simulink model "rcmodel"  (R2024b)
settings: Solver=FixedStepAuto  StartTime=0.0  StopTime=3500  FixedStep=0.1  RelTol=1e-3
undefined symbols (not defined in the file): ocv_interp, soc_target
libraries: fl_lib x8, nesl_utility x5, spspowerguiLib x1
settings Model: Creator=Acer  LastModifiedBy=Acer

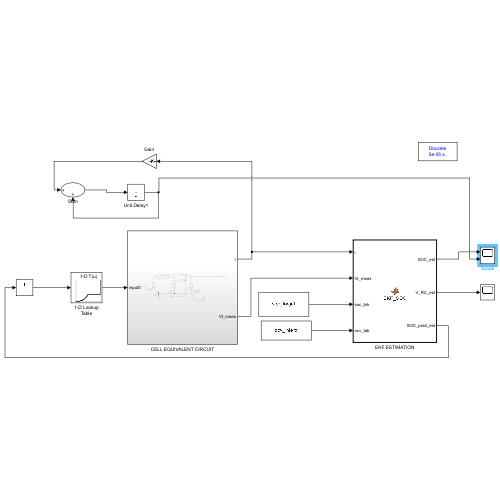
[thumbnail: Simulink's stored preview of the top-level diagram]
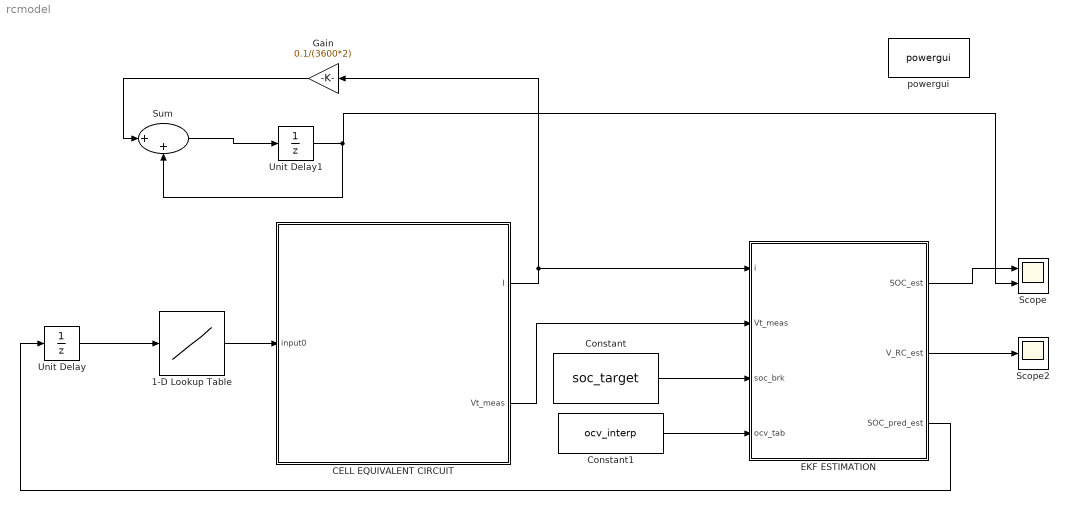
== system rcmodel ==
  1-D Lookup Table : Lookup_n-D  NumberOfTableDimensions=1  BreakpointsForDimension1=soc_target  Table=ocv_interp  ExtrapMethod=Clip  InternalRulePriority=Speed  RndMeth=Simplest
  CELL EQUIVALENT CIRCUIT : Subsystem
  Constant : Constant  Value=soc_target  SampleTime=0.1
  Constant1 : Constant  Value=ocv_interp  SampleTime=0.1
  EKF ESTIMATION : MATLAB Function  TreatAsAtomicUnit=on
  Gain : Gain  Gain=0.1/(3600*2)
  Scope : Scope  NumInputPorts=2
  Scope2 : Scope
  Sum : Sum  Inputs=|++
  Unit Delay : UnitDelay  InitialCondition=1  SampleTime=0.1  HasFrameUpgradeWarning=on
  Unit Delay1 : UnitDelay  InitialCondition=1  SampleTime=-1  HasFrameUpgradeWarning=on
  powergui : spspowerguiLib/powergui  Priority=1  SimulationMode=Discrete  SampleTime=50e-6  frequency=60  Iterations=50  frequencyindice=0  Pbase=100e6  ErrMax=1e-4  UnitsV=kV  UnitsW=MW  buscounter=0  FunctionMessages=off  echomessages=off  EnableUseOfTLC=off  CurrentSourceSwitches=off  DisableSnubberDevices=off  DisableRonSwitches=off  DisableVfSwitches=off  DisplayEquations=off  AutomaticDiscreteSolvers=off  SolverType=Tustin/Backward Euler (TBE)  Interpol=off  ExternalGateDelay=off  methode=off  Ts=100  x0status=blocks  SPID=on  SwTol=0  HookPort=off  NonlinearTolerance=1e-4  nMaxIteration=100  ContinueOnMaxIteration=off  RestoreLinks=warning  ResistiveCurrentMeasurement=off  Frange=[0:2:500]  Ylog=off  Xlog=on  ShowGrid=off  save=off  variable=ZData  structure=0  ZoomFFT=off  StartTime=0.0  cycles=1  DisplayStyle=1  fundamental=60  FreqAxis=off  MaxFrequency=1000  frequencyindicesteady=1  RmsSteady=1  display=off
  wires:
  Constant/1 -> EKF ESTIMATION/3(soc_brk)
  Constant1/1 -> EKF ESTIMATION/4(ocv_tab)
  EKF ESTIMATION/2(V_RC_est) -> Scope2/1
  Unit Delay1/1 -> Scope/2, Sum/2
  EKF ESTIMATION/1(SOC_est) -> Scope/1
  Unit Delay/1 -> 1-D Lookup Table/1
  EKF ESTIMATION/3(SOC_pred_est) -> Unit Delay/1
  Sum/1 -> Unit Delay1/1
  Gain/1 -> Sum/1
  CELL EQUIVALENT CIRCUIT/1(I) -> Gain/1, EKF ESTIMATION/1(i)
  1-D Lookup Table/1 -> CELL EQUIVALENT CIRCUIT/1(input0)
  CELL EQUIVALENT CIRCUIT/2(Vt_meas) -> EKF ESTIMATION/2(Vt_meas)

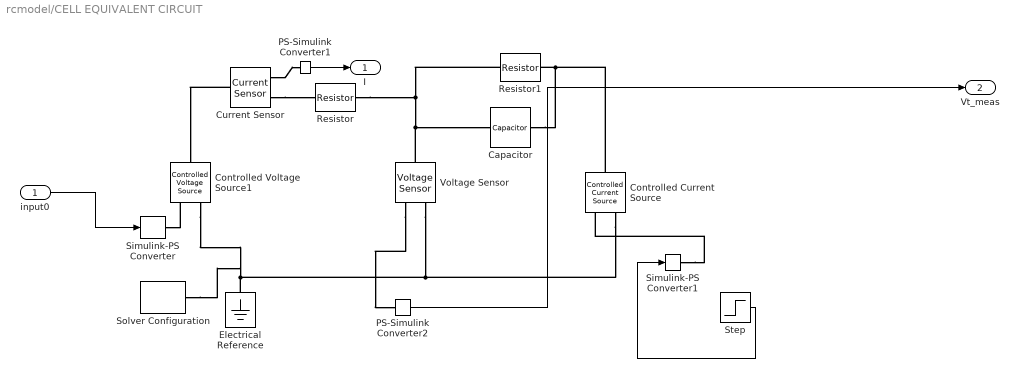
== system rcmodel/CELL EQUIVALENT CIRCUIT ==
  input0 : Inport
  Capacitor : fl_lib/Electrical/Electrical Elements/Capacitor  c=540 F  r=0 Ohm  g=0 1/Ohm  i_specify=off  i_priority=None  i=0 A  i_nominal_specify=off  i_nominal_value=1  i_nominal_unit=A  v_specify=off  v_priority=None  v=0 V  v_nominal_specify=off  v_nominal_value=1  v_nominal_unit=V  vc_specify=off  vc_priority=High  vc=0 V  vc_nominal_specify=off  vc_nominal_value=1  vc_nominal_unit=V
  Controlled Current Source : fl_lib/Electrical/Electrical Sources/Controlled Current Source
  Controlled Voltage Source1 : fl_lib/Electrical/Electrical Sources/Controlled Voltage Source
  Current Sensor : fl_lib/Electrical/Electrical Sensors/Current Sensor
  Electrical Reference : fl_lib/Electrical/Electrical Elements/Electrical Reference
  PS-Simulink Converter1 : nesl_utility/PS-Simulink Converter  PhysicalDomain=network_engine_domain  SubClassName=ps_output  LeftPortType=input  RightPortType=output  PseudoPeriodic=off  Frequencies=[]  VectorFormat=1-D array  Unit=A  AffineConversion=off
  PS-Simulink Converter2 : nesl_utility/PS-Simulink Converter  PhysicalDomain=network_engine_domain  SubClassName=ps_output  LeftPortType=input  RightPortType=output  PseudoPeriodic=off  Frequencies=[]  VectorFormat=1-D array  Unit=V  AffineConversion=off
  Resistor : fl_lib/Electrical/Electrical Elements/Resistor  R=0.149 Ohm  i_specify=off  i_priority=None  i=0 A  i_nominal_specify=off  i_nominal_value=1  i_nominal_unit=A  v_specify=off  v_priority=None  v=0 V  v_nominal_specify=off  v_nominal_value=1  v_nominal_unit=V
  Resistor1 : fl_lib/Electrical/Electrical Elements/Resistor  R=0.037 Ohm  i_specify=off  i_priority=None  i=0 A  i_nominal_specify=off  i_nominal_value=1  i_nominal_unit=A  v_specify=off  v_priority=None  v=0 V  v_nominal_specify=off  v_nominal_value=1  v_nominal_unit=V
  Simulink-PS Converter : nesl_utility/Simulink-PS Converter  PhysicalDomain=network_engine_domain  SubClassName=ps_input  LeftPortType=input  RightPortType=output  PseudoPeriodic=off  Frequencies=[]  NoiseDistribution=none  NoiseParameters=[]  Unit=1  AffineConversion=off  FilteringAndDerivatives=provide  SimscapeFilterOrder=1  InputFilterTimeConstant=0.001  UdotUserProvided=0
  Simulink-PS Converter1 : nesl_utility/Simulink-PS Converter  PhysicalDomain=network_engine_domain  SubClassName=ps_input  LeftPortType=input  RightPortType=output  PseudoPeriodic=off  Frequencies=[]  NoiseDistribution=none  NoiseParameters=[]  Unit=1  AffineConversion=off  FilteringAndDerivatives=provide  SimscapeFilterOrder=1  InputFilterTimeConstant=0.001  UdotUserProvided=0
  Solver Configuration : nesl_utility/Solver Configuration  PhysicalDomain=network_engine_domain  SubClassName=solver  LeftPortType=input  RightPortType=generic  Tones=[]  Harmonics=[]  SimulateNoise=off  Profile=off  UseLocalSampling=off  EnableSwitchedLinearOptims=on  FrequencyDomain=off  UseCCode=off  RelTol=0.001  AbsTol=0.001  MinStep=1e-09  ToWorkspace=off  RevertToSquareIcSolve=off  NumHomotopyIterations=100  PhasorMode=off  PhasorModeNumHarmonics=1  ConsistencySolver=NEWTON_XTOL_AFTER_FTOL  IndexReductionMethod=DerivativeReplacement  DoDC=off  ResidualTolerance=1e-09  ConsistencyTolSource=GLOBAL  ConsistencyAbsTol=0.001  ConsistencyRelTol=0.001  ConsistencyTolFactor=0.001  UseLocalSolver=off  LocalSolverChoice=NE_BACKWARD_EULER_ADVANCER  ResolveIndetEquations=on  FunctionEvalNumThread=1  LocalSolverSampleTime=0.001  DoFixedCost=off  MaxNonlinIter=3  MaxModeIter=2  ComputeImpulses=off  ImpulseIterations=2  LinearAlgebra=auto  LinearAlgebraNumThread=0  EquationFormulation=NE_TIME_EF  DelaysMemoryBudget=1024  AutomaticFiltering=on  FilteringTimeConstant=0.001  PartitionStorageMethod=AS_NEEDED  PartitionMemoryBudget=1024  PartitionMethod=ROBUST  MultibodyUseLocalSolver=off  MultibodyLocalSolverChoice=ODE1  MultibodyLocalSolverSampleTime=0.001
  Step : Step  Time=-1  SampleTime=0
  Voltage Sensor : fl_lib/Electrical/Electrical Sensors/Voltage Sensor
  I : Outport
  Vt_meas : Outport  Port=2
  wires:
  Step/1 -> Simulink-PS Converter1/1
  PS-Simulink Converter2/1 -> Vt_meas/1
  input0/1 -> Simulink-PS Converter/1
  PS-Simulink Converter1/1 -> I/1
  connections:
  Voltage Sensor/RConn2 -- Solver Configuration/RConn1 -- Controlled Voltage Source1/RConn2 -- Electrical Reference/LConn1 -- Controlled Current Source/RConn2
  Simulink-PS Converter1/RConn1 -- Controlled Current Source/RConn1
  Simulink-PS Converter/RConn1 -- Controlled Voltage Source1/RConn1
  Resistor1/LConn1 -- Voltage Sensor/LConn1 -- Capacitor/LConn1 -- Resistor/RConn1
  Voltage Sensor/RConn1 -- PS-Simulink Converter2/LConn1
  Current Sensor/RConn2 -- Resistor/LConn1
  Current Sensor/RConn1 -- PS-Simulink Converter1/LConn1
  Current Sensor/LConn1 -- Controlled Voltage Source1/LConn1
  Capacitor/RConn1 -- Controlled Current Source/LConn1 -- Resistor1/RConn1

== matlab function rcmodel/EKF ESTIMATION ==
  settings: updateMethod=DISCRETE  sampleTime=0.1
  data: i input size=1; SOC_est output size=1; Vt_meas input size=1; V_RC_est output size=1; soc_brk input; ocv_tab input; SOC_pred_est output
function [SOC_est, V_RC_est, SOC_pred_est] = EKF_SOC(i, Vt_meas, soc_brk, ocv_tab)
% EKF for SOC estimation with 1st-order RC model
% Outputs:
%   SOC_est      - corrected SOC (after EKF correction)
%   V_RC_est     - estimated RC voltage
%   SOC_pred_est - predicted SOC (before correction) - for breaking algebraic loop

% Persistent state, covariance, and derivative table
persistent x_hat P docv_tab
if isempty(x_hat)
    x_hat = [1; 0];                % initial SOC = 1, V_RC = 0
    P = diag([0.01, 0.01]);        % initial uncertainty
    docv_tab = gradient(ocv_tab, soc_brk);
end

% Battery parameters
Q_nom = 2;          % Ah
R0 = 0.149;         % ohm
R1 = 0.037;         % ohm
C1 = 540;           % F
tau = R1 * C1;
Delta_t = 0.1;

% Noise covariances
Q = diag([1e-5, 1e-4]);
R = 1e-3;

% ----- Prediction -----
x_pred = x_hat;
% SOC update (Coulomb counting)
x_pred(1) = x_hat(1) + (Delta_t / (3600 * Q_nom)) * i;
% RC voltage update
x_pred(2) = exp(-Delta_t/tau) * x_hat(2) + R1 * (1 - exp(-Delta_t/tau)) * i;

% Save predicted SOC for output (to feed lookup table)
SOC_pred_est = x_pred(1);

% State transition matrix and covariance prediction
A = [1, 0; 0, exp(-Delta_t/tau)];
P_pred = A * P * A' + Q;

% ----- Linearisation -----
dOCV = interp1(soc_brk, docv_tab, x_pred(1), 'linear', 'extrap');

H = [dOCV, -1];

% ----- Kalman gain -----
S = H * P_pred * H' + R;
K = P_pred * H' / S;

% ----- Correction -----
OCV_pred = interp1(soc_brk, ocv_tab, x_pred(1), 'linear', 'extrap');
Vt_pred = OCV_pred - x_pred(2) - i * R0;
innovation = Vt_meas - Vt_pred;
x_new = x_pred + K * innovation;

% ----- Covariance update -----
P_new = (eye(2) - K * H) * P_pred;

% ----- Update persistent variables -----
x_hat = x_new;
P = P_new;

% ----- Outputs -----
SOC_est = x_hat(1);
V_RC_est = x_hat(2);

end
